simulink model "TP3_simu_realim_obs_discreto"  (R2023b)
settings: Solver=VariableStepAuto  StartTime=0.0  StopTime=10  FixedStep=20e-3  RelTol=1e-3
values from neighbouring files (symbols this model uses):
  A = sysc .A    [Prueba_Control.m]
  Ad = sysd .A    [Prueba_Control.m]    (also in Prueba_Control_CI.m = sysd.A; control3.m = sysd.A)
  B = sysc .B    [Prueba_Control.m]
  Bd = sysd .B    [Prueba_Control.m]    (also in Prueba_Control_CI.m = sysd.B; control3.m = sysd.B)
  C = sysc .C    [Prueba_Control.m]
  Cd = sysd .C    [Prueba_Control.m]    (also in Prueba_Control_CI.m = sysd.C; control3.m = sysd.C)
  Kd = acker (Ad , Bd , polyd )    [Prueba_Control.m]    (also in Prueba_Control_CI.m = place(Ad,Bd,polesd_ctrl); control3.m = place(Ad,Bd,polesd_ctrl))
  Ld = acker (Ad.', Cd.', polyed ).'    [Prueba_Control.m]    (also in Prueba_Control_CI.m = place(Ad', Cd',polesd_obs)'; control3.m = place(Ad', Cd',polesd_obs).')
  Ts = 0.02    [Guardado_de_datos_TP3.m]    (also in Prueba_Control.m; Prueba_Control_CI.m; control3.m; registro_175533.mat)
  x1e = 0    [Prueba_Control_CI.m]    (also in control3.m)
  x2e = 0    [Prueba_Control_CI.m]    (also in control3.m)
  x3e = 0    [Prueba_Control_CI.m]    (also in control3.m)
  x4e = 0    [Prueba_Control_CI.m]    (also in control3.m)
settings Model: Creator=manuh  LastModifiedBy=ApoloXVIII

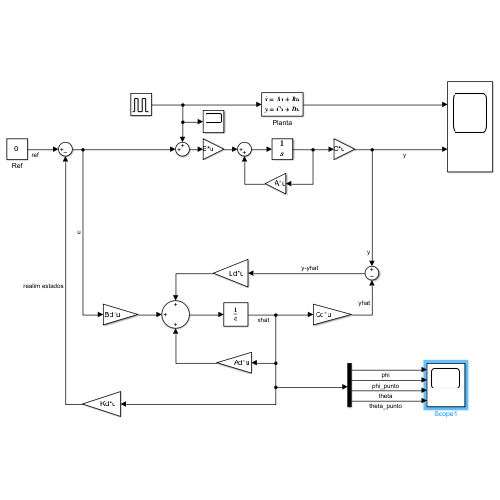
[thumbnail: Simulink's stored preview of the top-level diagram]
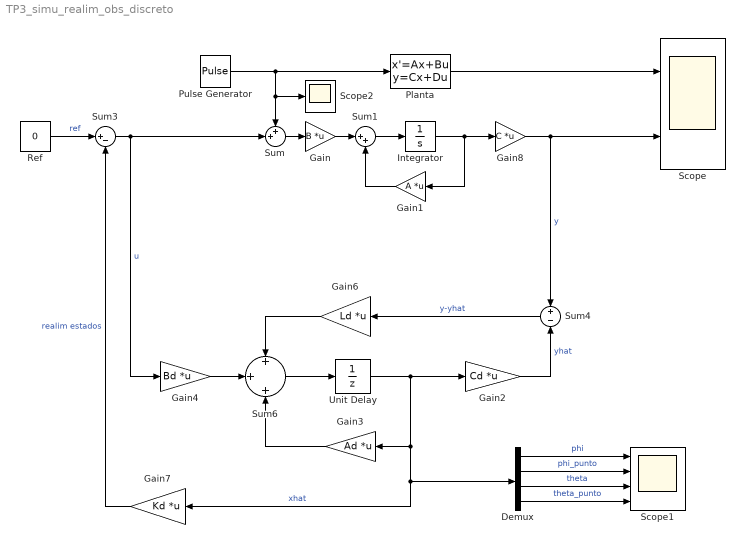
== system TP3_simu_realim_obs_discreto ==
  Demux : Demux
  Gain : Gain  Gain=B  Multiplication=Matrix(K*u)
  Gain1 : Gain  Gain=A  Multiplication=Matrix(K*u)
  Gain2 : Gain  Gain=Cd  Multiplication=Matrix(K*u)
  Gain3 : Gain  Gain=Ad  Multiplication=Matrix(K*u)
  Gain4 : Gain  Gain=Bd  Multiplication=Matrix(K*u)
  Gain6 : Gain  Gain=Ld  Multiplication=Matrix(K*u)
  Gain7 : Gain  Gain=Kd  Multiplication=Matrix(K*u)
  Gain8 : Gain  Gain=C  Multiplication=Matrix(K*u)
  Integrator : Integrator
  Planta : StateSpace  A=A  B=B  C=C  D=0  InitialCondition=[x1e,x2e,x3e,x4e]
  Pulse Generator : DiscretePulseGenerator  PulseType=Time based  Amplitude=-20  Period=30  PulseWidth=0.1  PhaseDelay=3
  Ref : Constant  Value=0
  Scope : Scope  NumInputPorts=2
  Scope1 : Scope  NumInputPorts=4
  Scope2 : Scope
  Sum : Sum  Inputs=++|
  Sum1 : Sum  Inputs=|++
  Sum3 : Sum  Inputs=|+-
  Sum4 : Sum  Inputs=+|-
  Sum6 : Sum  Inputs=+|+|+
  Unit Delay : UnitDelay  InitialCondition=[x1e,x2e,x3e,x4e]  SampleTime=Ts  HasFrameUpgradeWarning=on
  wires:
  Ref/1 -> Sum3/1  "ref"
  Sum3/1 -> Gain4/1, Sum/2  "u"
  Sum4/1 -> Gain6/1  "y-yhat"
  Gain2/1 -> Sum4/2  "yhat"
  Unit Delay/1 -> Gain2/1, Demux/1, Gain7/1, Gain3/1  "xhat"
  Gain3/1 -> Sum6/3
  Sum6/1 -> Unit Delay/1
  Gain4/1 -> Sum6/2
  Gain6/1 -> Sum6/1
  Gain7/1 -> Sum3/2  "realim estados"
  Demux/1 -> Scope1/1  "phi"
  Demux/2 -> Scope1/2  "phi_punto"
  Demux/3 -> Scope1/3  "theta"
  Demux/4 -> Scope1/4  "theta_punto"
  Pulse Generator/1 -> Scope2/1, Sum/1, Planta/1
  Planta/1 -> Scope/1
  Sum1/1 -> Integrator/1
  Gain1/1 -> Sum1/2
  Sum/1 -> Gain/1
  Gain/1 -> Sum1/1
  Gain8/1 -> Sum4/1, Scope/2  "y"
  Integrator/1 -> Gain1/1, Gain8/1
